simulink library "runningAverage_cl"  (R2018a)
settings: Solver=VariableStepAuto  StartTime=0.0  StopTime=10.0  RelTol=1e-3
libraries: resettableTimer_ul x1
settings Model: Creator=mcobb  LastModifiedBy=mcobb

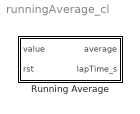
== system runningAverage_cl ==
  Running Average : Subsystem

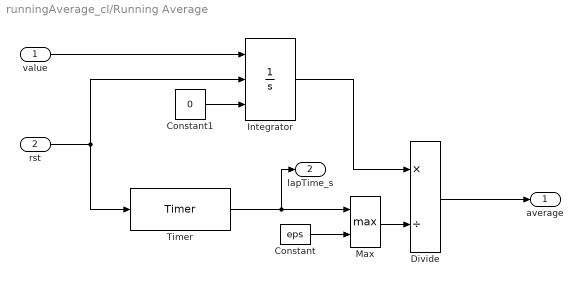
== system runningAverage_cl/Running Average ==
  value : Inport
  rst : Inport  Port=2
  Constant : Constant  Value=eps
  Constant1 : Constant  Value=0
  Divide : Product  Inputs=*/
  Integrator : Integrator  ExternalReset=rising  InitialConditionSource=external
  Max : MinMax  Function=max  Inputs=2
  Timer : resettableTimer_ul/Timer
  average : Outport
  lapTime_s : Outport  Port=2
  wires:
  Timer/1 -> lapTime_s/1, Max/1
  Constant/1 -> Max/2
  Max/1 -> Divide/2
  value/1 -> Integrator/1
  rst/1 -> Timer/1, Integrator/2
  Constant1/1 -> Integrator/3
  Integrator/1 -> Divide/1
  Divide/1 -> average/1
